simulink model "muckabout"  (R2021a)
settings: Solver=FixedStepAuto  StartTime=0.0  StopTime=860  FixedStep=0.005  RelTol=1e-3
libraries: fl_lib x6, nesl_utility x4
settings Model: Creator=Henry  LastModifiedBy=Henry

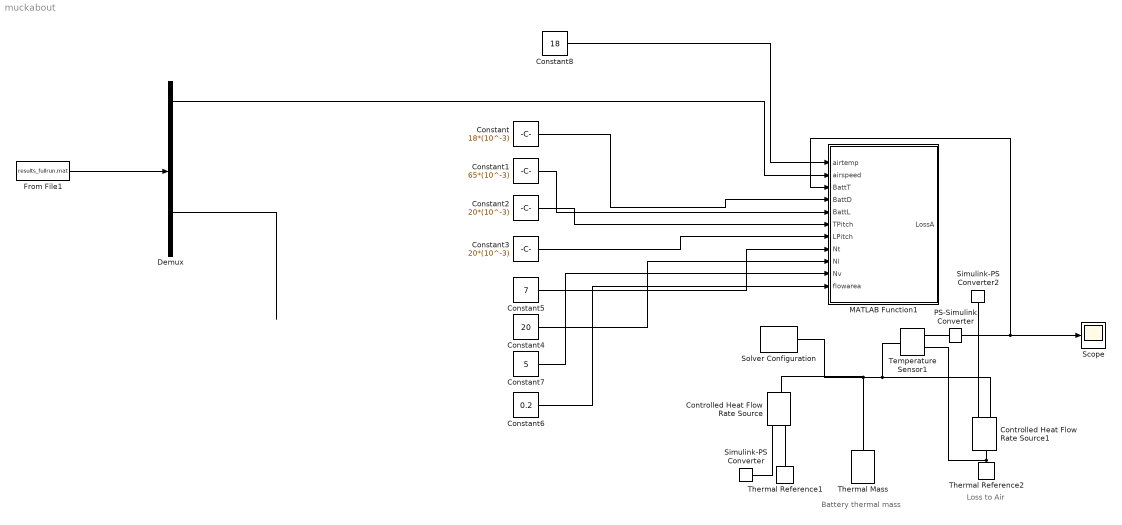
== system muckabout ==
  note: Loss to Air
  note: Battery thermal mass
  Constant : Constant  Value=18*(10^-3)
  Constant1 : Constant  Value=65*(10^-3)
  Constant2 : Constant  Value=20*(10^-3)
  Constant3 : Constant  Value=20*(10^-3)
  Constant4 : Constant  Value=20
  Constant5 : Constant  Value=7
  Constant6 : Constant  Value=0.2
  Constant7 : Constant  Value=5
  Constant8 : Constant  Value=18
  Controlled Heat Flow Rate Source : fl_lib/Thermal/Thermal Sources/Controlled Heat Flow Rate Source
  Controlled Heat Flow Rate Source1 : fl_lib/Thermal/Thermal Sources/Controlled Heat Flow Rate Source
  Demux : Demux  Outputs=12
  From File1 : FromFile  FileName=results_fullrun.mat  SampleTime=0
  MATLAB Function1 : MATLAB Function  TreatAsAtomicUnit=on
  PS-Simulink Converter : nesl_utility/PS-Simulink Converter  PhysicalDomain=network_engine_domain  SubClassName=ps_output  LeftPortType=input  RightPortType=output  PseudoPeriodic=off  Frequencies=[]  Unit=inherit  AffineConversion=off
      settings: SourceProductBaseCode=PW,SS
  Scope : Scope
  Simulink-PS Converter : nesl_utility/Simulink-PS Converter  PhysicalDomain=network_engine_domain  SubClassName=ps_input  LeftPortType=input  RightPortType=output  PseudoPeriodic=off  Frequencies=[]  NoiseDistribution=none  NoiseParameters=[]  Unit=1  AffineConversion=off  FilteringAndDerivatives=provide  SimscapeFilterOrder=1  InputFilterTimeConstant=0.001  UdotUserProvided=0
      settings: SourceProductBaseCode=PW,SS
  Simulink-PS Converter2 : nesl_utility/Simulink-PS Converter  PhysicalDomain=network_engine_domain  SubClassName=ps_input  LeftPortType=input  RightPortType=output  PseudoPeriodic=off  Frequencies=[]  NoiseDistribution=none  NoiseParameters=[]  Unit=1  AffineConversion=off  FilteringAndDerivatives=provide  SimscapeFilterOrder=1  InputFilterTimeConstant=0.001  UdotUserProvided=0
      settings: SourceProductBaseCode=PW,SS
  Solver Configuration : nesl_utility/Solver Configuration  PhysicalDomain=network_engine_domain  SubClassName=solver  LeftPortType=input  RightPortType=generic  Tones=[]  Harmonics=[]  SimulateNoise=off  Profile=off  UseLocalSampling=off  EnableSwitchedLinearOptims=on  FrequencyDomain=off  UseCCode=off  RelTol=0.001  AbsTol=1e-06  MinStep=1e-09  ToWorkspace=off  RevertToSquareIcSolve=off  NumHomotopyIterations=100  PhasorMode=off  PhasorModeNumHarmonics=1  DoDC=off  ResidualTolerance=1e-09  UseLocalSolver=off  LocalSolverChoice=NE_BACKWARD_EULER_ADVANCER  LocalSolverSampleTime=0.001  DoFixedCost=off  MaxNonlinIter=3  MaxModeIter=2  ComputeImpulses=off  ImpulseIterations=2  LinearAlgebra=auto  EquationFormulation=NE_TIME_EF  DelaysMemoryBudget=2048  AutomaticFiltering=on  FilteringTimeConstant=0.001  PartitionStorageMethod=AS_NEEDED  PartitionMemoryBudget=1024  PartitionMethod=ROBUST
      settings: SourceProductBaseCode=PW,SS
  Temperature Sensor1 : fl_lib/Thermal/Thermal Sensors/Temperature Sensor
  Thermal Mass : fl_lib/Thermal/Thermal Elements/Thermal Mass  mass=100 kg  sp_heat=1000 J/kg/K  T_specify=on  T_priority=High  T=300 K  T_nominal_specify=off  T_nominal_unit=K  T_nominal_value=1  Q_specify=off  Q_priority=None  Q=0 W  Q_nominal_specify=off  Q_nominal_unit=W  Q_nominal_value=1
  Thermal Reference1 : fl_lib/Thermal/Thermal Elements/Thermal Reference
  Thermal Reference2 : fl_lib/Thermal/Thermal Elements/Thermal Reference
  wires:
  From File1/1 -> Demux/1
  Constant7/1 -> MATLAB Function1/10(Nv)
  Constant6/1 -> MATLAB Function1/11(flowarea)
  Constant4/1 -> MATLAB Function1/9(Nl)
  Constant3/1 -> MATLAB Function1/7(LPitch)
  Constant1/1 -> MATLAB Function1/5(BattL)
  Constant5/1 -> MATLAB Function1/8(Nt)
  Constant/1 -> MATLAB Function1/4(BattD)
  Demux/1 -> MATLAB Function1/2(airspeed)
  Constant2/1 -> MATLAB Function1/6(TPitch)
  PS-Simulink Converter/1 -> Scope/1, MATLAB Function1/3(BattT)
  Constant8/1 -> MATLAB Function1/1(airtemp)
  Demux/10 -> ?
  connections:
  Controlled Heat Flow Rate Source1/RConn2 -- Temperature Sensor1/LConn1 -- Solver Configuration/RConn1 -- Controlled Heat Flow Rate Source/LConn1 -- Thermal Mass/LConn1
  Thermal Reference2/LConn1 -- Temperature Sensor1/RConn1 -- Controlled Heat Flow Rate Source1/LConn1
  Controlled Heat Flow Rate Source1/RConn1 -- Simulink-PS Converter2/RConn1
  Controlled Heat Flow Rate Source/RConn2 -- Thermal Reference1/LConn1
  Controlled Heat Flow Rate Source/RConn1 -- Simulink-PS Converter/RConn1
  PS-Simulink Converter/LConn1 -- Temperature Sensor1/RConn2

== matlab function muckabout/MATLAB Function1 ==
  data: airtemp input; airspeed input; BattT input; BattD input; LossA output; BattL input; TPitch input; LPitch input; Nt input; Nl input; Nv input; flowarea input
function LossA  = Battfcn(airtemp,airspeed,BattT,BattD,BattL,TPitch,LPitch,Nt,Nl,Nv,flowarea)

T = [250,275,300,325,350]-273.15;
mu = [1.599,1.725,1.846,1.962,2.075].*(10^-5);
rho = [1.412,1.284,1.177,1.086,1.009];

rho = interp1(T,rho,airtemp);
dm = flowarea*airspeed*rho;

 %Fmax = dm*airspeed;         %maximum force the air could exert on the battery air intake
 %Pmax = Fmax/flowarea;       %maximum guage pressure possible at air intake
Pmax = 0.5*rho*(airspeed^2);

mufs = interp1(T,mu,airtemp);
mus = interp1(T,mu,BattT);

filmT1 = (BattT + airtemp)/2;

[ReN,PrN,GrN,kN,CpaN] = Variablefinder('air',filmT1,airtemp,0,BattL*Nv);     %cells are verticaly oriented so the natural convection parameters are found using height not diameter

[Re,Pr,Gr,k,Cpa] = Variablefinder('air',filmT1,airtemp,airspeed,BattD);
for x = 1:5
    fric = (0.44 + (0.08*LPitch/BattD)/(((TPitch-BattD)/BattD)^(0.43+1.13*(BattD/LPitch))))*Re^(-0.15);     %friction coefficient for in-line pack
    Gmax = ( ((Pmax)*rho) / (2*fric*Nt*Nv*((mus/mufs)^0.14)) )^(1/2);          %maximum masss flow rate through battery based on max pressure at intake
    umax = (Gmax/(flowarea*rho))*(TPitch/(TPitch-BattD));                   %peak air speed within pack
    [Re,Pr,Gr,k,Cpa] = Variablefinder('air',filmT1,airtemp,umax,BattD);     %re-find variables based on speed
end

if Gmax > dm
    Gmax = dm;
    umax = (Gmax/(flowarea*rho))*(TPitch/(TPitch-BattD));                   %peak air speed within pack
    [Re,Pr,Gr,k,Cpa] = Variablefinder('air',filmT1,airtemp,umax,BattD);     %re-find variables based on speed
end

[Res,Prs,Grs,ks,Cps] = Variablefinder('air',BattT,BattT,umax,BattD);

if GrN/(Re^2) < 1
    if Re < 100
        C1 = 0.9;
        m = 0.4;
        n = 0.36;
    elseif Re < 1000
        C1 = 0.52;
        m = 0.5;
        n = 0.36;
    elseif Re < (2*(10^5))
        C1 = 0.27;
        m = 0.63;
        n = 0.36;
    else
        C1 = 0.033;
        m = 0.8;
        n = 0.4;
    end
C2 = 1;
    switch Nl
        case (1)
            C2 = 0.7;    
        case (2)
            C2 = 0.8;
        case (3)
            C2 = 0.86;
        case (4)
            C2 = 0.9;
        case (5)
            C2 = 0.92;
        case(7)
            C2 = 0.95;
        case(10)
            C2 = 0.97;
        case(13)
            C2 = 0.98;
        case(16)
            C2 = 0.99;
        case(20)
            C2 = 1;
    end

    Nu = C2*C1*(Re^m)*(Pr^n)*((Pr/Prs)^0.25);
    
    h = Nu*k/(BattD);
    R = 1/( (Nt*Nv*Nl*BattD*pi()*BattL) * h );
    
    airout = BattT - (BattT-airtemp)*exp(-1/(Gmax*Cpa*R));        %(h*(Nt*Nl*BattD*pi()*BattL))
    %airout = ( BattT + ((Gmax*Cpa*R) - 1/2)*airtemp ) / ((Gmax*Cpa*R) + 1/2);
    LossA = Gmax*Cpa*(airout-airtemp);
else
    Ra = PrN*GrN;  %calculate the rayleigh number
    Nu = (0.68 + ( (0.387*(Ra^(1/6))) / ((1 + ((0.492/PrN)^(9/16)))^(8/27)) ) )^2;
    %Nu = 0.478*(GrN^0.25);
    
    h = Nu*k/(BattL*Nv);
    R = 1/( (Nt*Nv*Nl*BattD*pi()*BattL) * h );
    LossA = (BattT-((airtemp+BattT)/2))/R;
end

end
